simulink model "DiscretePulseGenerator_TestGen6"  (R2017b)
settings: Solver=FixedStepDiscrete  StartTime=0.0  StopTime=10.0  RelTol=1e-3
undefined symbols (not defined in the file): Block_TestLib, enable
settings Model: Creator=hbourbou  LastModifiedBy=hbourbou
settings DebuggingCC: ParameterOverflowMsg=none

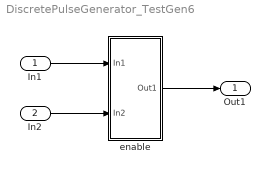
== system DiscretePulseGenerator_TestGen6 ==
  In1 : Inport
  In2 : Inport  Port=2
  enable : Subsystem  AncestorBlock=Block_TestLib/enable
  Out1 : Outport
  wires:
  In1/1 -> enable/1(In1)
  In2/1 -> enable/2(In2)
  enable/1(Out1) -> Out1/1

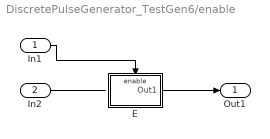
== system DiscretePulseGenerator_TestGen6/enable ==
  In1 : Inport  OutDataTypeStr=boolean
  In2 : Inport  Port=2
  E : Subsystem  TreatAsAtomicUnit=on
  Out1 : Outport
  wires:
  In1/1 -> E/Enable
  In2/1 -> ?
  E/1(Out1) -> Out1/1

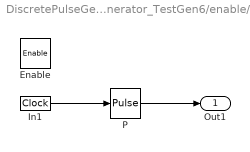
== system DiscretePulseGenerator_TestGen6/enable/E ==
  Enable : EnablePort
  In1 : DigitalClock  SampleTime=0.1
  P : DiscretePulseGenerator  TimeSource=Use external signal  Amplitude=0.5  Period=5  PulseWidth=3  SampleTime=-1
  Out1 : Outport
  wires:
  In1/1 -> P/1
  P/1 -> Out1/1
